simulink model "aero"  (R2021b)
settings: Solver=VariableStepAuto  StartTime=0.0  StopTime=10.0  RelTol=1e-3
libraries: aerodynamics x1, coordinate_transforms x1
settings Model: Creator=Nikita  LastModifiedBy=Nikita

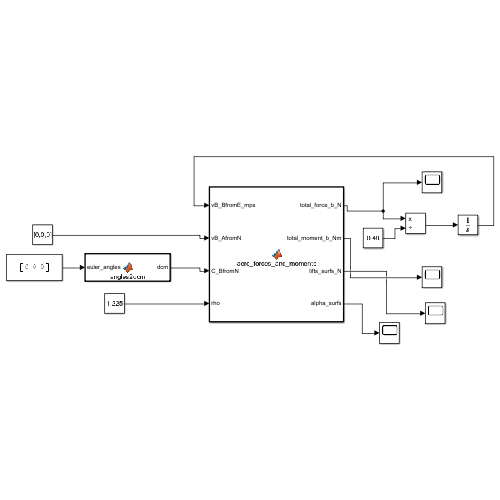
[thumbnail: Simulink's stored preview of the top-level diagram]
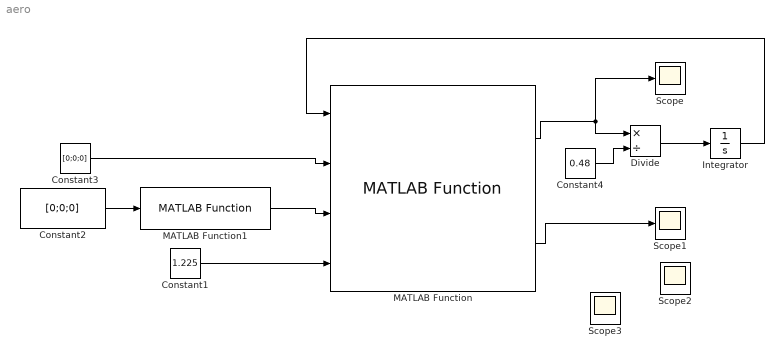
== system aero ==
  Constant1 : Constant  Value=1.225
  Constant2 : Constant  Value=[0;0;0]
  Constant3 : Constant  Value=[0;0;0]
  Constant4 : Constant  Value=0.48
  Divide : Product  Inputs=*/
  Integrator : Integrator  InitialCondition=[100;0;0];
  MATLAB Function : aerodynamics/MATLAB Function  SystemSampleTime=-1  VariantActivationTime=update diagram  Latency=0  AutoFrameSizeCalculation=off
  MATLAB Function1 : coordinate_transforms/MATLAB Function  SystemSampleTime=-1  VariantActivationTime=update diagram  Latency=0  AutoFrameSizeCalculation=off
  Scope{,1..3} (4 alike) : Scope
  wires:
  MATLAB Function/1 -> Divide/1, Scope/1
  MATLAB Function/2 -> Scope1/1
  Integrator/1 -> MATLAB Function/1
  Constant1/1 -> MATLAB Function/4
  MATLAB Function1/1 -> MATLAB Function/3
  Constant2/1 -> MATLAB Function1/1
  Constant3/1 -> MATLAB Function/2
  Constant4/1 -> Divide/2
  Divide/1 -> Integrator/1
  ? -> Scope2/1
  ? -> Scope3/1
